simulink model "shoot2"  (R2017b)
settings: Solver=VariableStepAuto  StartTime=0.0  StopTime=10.0  RelTol=1e-3
settings Model: Creator=ghleila  LastModifiedBy=ghleila

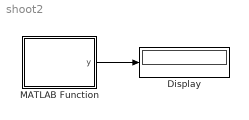
== system shoot2 ==
  Display : Display
  MATLAB Function : MATLAB Function  TreatAsAtomicUnit=on
  wires:
  MATLAB Function/1(y) -> Display/1

== matlab function shoot2/MATLAB Function ==
  data: y output; A data_store_memory
function y = fcn
%#codegen
global U;
U = U+1;
y = U;
